simulink model "VFlexP"  (R2025a)
settings: Solver=ode23tb  StartTime=0.0  StopTime=40  FixedStep=5e-5
model workspace (MAT data in the model file):
  DCop_DCBUCK : object (value not decoded)
  Grid_CCVSC_idx = [2; 3; 4; 5; 6; 7; 8; 9; 10; 11; 12]
  Grid_CCVSCs = 1
  Grid_CCVSCs_buses = 1
  Grid_CCVSCs_toM = [0 1 0 0 0 0 0 0 0 0 0 0 ... (781 elements, 71x11)]
  Grid_C_Lines = [0.1 0.1 0.1 0.1]
  Grid_Cbuses = [0.05000002 0.10000002 0.10000002 0.10000002 0.05000002]
  Grid_DC : object (value not decoded)
  Grid_DCop_DCBUCK : object (value not decoded)
  Grid_DCop_DC_PES : object (value not decoded)
  Grid_DFIGs = 1
  Grid_DFIGs_buses = 1
  Grid_DGs : string (value not decoded)
  Grid_From_buses = [1 2 4 4]
  Grid_GFls = 1
  Grid_GFls_buses = 1
  Grid_GFr_idx = [1; 2; 3]
  Grid_GFrs = 1
  Grid_GFrs_buses = 1
  Grid_GFrs_toM = [1 0 0 0 0 0 0 0 0 1 0 0 ... (15 elements, 5x3)]
  Grid_IG_idx = 1
  Grid_IGs = 1
  Grid_IGs_buses = 1
  Grid_IGs_toM = [1; 0]
  Grid_L_Lines = [0.5 0.5 0.5 0.5]
  Grid_L_Loads = [0.000959999944704 0.000156249997559 0.00154855477548]
  Grid_Lines_fromM : object (value not decoded)
  Grid_Lines_toM : object (value not decoded)
  Grid_Load_buses = [2; 3; 4]
  Grid_Load_busesDC = []
  Grid_MGES_idx = [1; 2; 3]
  Grid_MGESs = 1
  Grid_MGESs_buses = [1; 5; 3]
  Grid_MGESs_toM = [1 0 0 0 0 0 0 0 0 1 0 0 ... (15 elements, 5x3)]
  Grid_MSGs = 1
  Grid_MSGs_buses = 1
  Grid_Nbuses = 5
  Grid_PQ_gen = [3; 2; 2]
  Grid_Ploads = [1250 4000 1250]
  Grid_PloadsDC = []
  Grid_Ps_lf = [0.274439537683 0.78 0.3]
  Grid_Qloads = [0.3 0.5 0.5]
  Grid_Qs_lf = [-0.0366071562958 0.126505596722 -0.0162964024532]
  Grid_R_Lines = [0.01 0.01 0.01 0.01]
  Grid_R_Loads = [3.9999997696 1.24999998047 3.8713869387]
  Grid_R_Loads_DC = 0
  Grid_Rcf = [50000000 50000000 50000000 50000000 50000000]
  Grid_SCs = 1
  Grid_SCs_buses = 1
  Grid_SG_idx = 1
  Grid_SGs = 1
  Grid_SGs_buses = 1
  Grid_SGs_toM = [1; 0]
  Grid_To_buses = [2 3 3 5]
  Grid_VCVSC_idx = [1; 2; 3; 4; 5; 6; 7; 8; 9; 10; 11; 12]
  Grid_VCVSCs = 1
  Grid_VCVSCs_buses = [1; 2; 3; 6; 8; 9; 12; 58; 59; 60; 63; 65]
  Grid_VCVSCs_toM = [1 0 0 0 0 0 0 0 0 0 0 0 ... (852 elements, 71x12)]
  Grid_VSM_idx = [1; 2; 3]
  Grid_VSMs = 1
  Grid_VSMs_buses = 1
  Grid_VSMs_toM = [1 0 0 0 0 0 0 0 0 1 0 0 ... (15 elements, 5x3)]
  Grid_admitt_matrix = [2.15353135314-19.7953135314i  -1.9801980198+19.801980198i; -1.9801980198+19.801980198i  2.15353135314-19.7953135314i]
  Grid_admitt_matrix_noloads = [1.98686468647-19.7953135314i  -1.9801980198+19.801980198i; -1.9801980198+19.801980198i  1.98686468647-19.7953135314i]
  Grid_bus = [1; 2; 6; 7; 8]
  Grid_busDC_complexity = [1 1 1]
  Grid_busDC_complexity_PF = [2 2 2]
  Grid_bus_complexity = [1 1 1 1 1]
  Grid_bus_complexity_PF = [1 1 1 1 1]
  Grid_buses_lf = [1; 5; 3]
  Grid_conductance_matrix = [100.00000002  -100  0; -100  200.00000002  -100; 0  -100  100.00000002]
  Grid_conductance_matrix_noloads = [100.00000002  -100  0; -100  200.00000002  -100; 0  -100  100.00000002]
  Grid_fref : object (value not decoded)
  Grid_gen_static_params : mBase (value not decoded)
  Grid_iPs_lf = [3.64378984326 1.28205128205 3.33333333333]
  Grid_iQs_lf = [-27.3170631425 7.90478860943 -61.3632366329]
  Grid_iadmitt_matrix = [2.88165849328-0.0982918688642i  2.87905051706-0.123273862303i; 2.87905051706-0.123273862303i  2.88165849328-0.0982918688642i]
  Grid_iadmitt_matrix_noloads = [37.5012524798-37.4874983544i  37.4987475202-37.5125016456i; 37.4987475202-37.5125016456i  37.5012524798-37.4874983544i]
  Grid_iconductance_matrix = [16666671.4556  16666671.4489  16666671.4456; 16666671.4489  16666671.4522  16666671.4489; 16666671.4456  16666671.4489  16666671.4556]
  Grid_iconductance_matrix_noloads = [16666671.4556  16666671.4489  16666671.4456; 16666671.4489  16666671.4522  16666671.4489; 16666671.4456  16666671.4489  16666671.4556]
  Grid_init_OK_bool = 1
  Grid_intconv_PF : object (value not decoded)
  Grid_lf_op : op_report (value not decoded)
  Grid_lineDC_complexity = [1 1]
  Grid_lineDC_complexity_PF = [2 2]
  Grid_line_complexity = [1 1 1 1]
  Grid_line_complexity_PF = [3 3 3 3]
  Grid_loadDC_complexity = []
  Grid_loadDC_complexity_PF = []
  Grid_load_complexity = [3 3 3]
  Grid_load_complexity_PF = [4 4 4]
  Grid_opDC_CCVSC : object (value not decoded)
  Grid_opDC_VSM : object (value not decoded)
  Grid_opGFr : object (value not decoded)
  Grid_opVCVSC : object (value not decoded)
  Grid_op_CCVSC : object (value not decoded)
  Grid_op_IG : object (value not decoded)
  Grid_op_MGES : object (value not decoded)
  Grid_op_SG : object (value not decoded)
  Grid_op_VSM : object (value not decoded)
  Grid_shift_lines = [0 0 0 0]
  Grid_tap_lines = [1 1 1 1]
  Grid_v_buses_mod = [1 1 1 0.9837920967 1]
  LinsysParamChangeStruct : Param1 (value not decoded)
  Lline = 0.01
  Rline = 1e-05
  linsys : object (value not decoded)
symbols that are objects in the model workspace (value not decoded): Grid_DCop_DC_PES, Grid_DCop_DCBUCK, Grid_op_CCVSC, Grid_op_IG, Grid_op_MGES, Grid_op_SG, Grid_op_VSM, Grid_opDC_CCVSC, Grid_opDC_VSM, Grid_opGFr, Grid_opVCVSC
undefined symbols (not defined in the file): block_buses_DC, block_idx, CCVSC_idx, Cf, costs, costs2, D, DFIGs_nodes, DiscIntNeverNeededParam, entity, Fb, Fi, From_nodes, grid_linsys, Grid_op_DFIG, Grid_op_DFIG_PQ, Grid_op_MSG, Grid_op_SC, Grid_op_VCVSC, H, initial_states_grid, K_1, K_3, K_5, K_A, K_C, K_IM, K_IR, K_P, K_PM, K_PR, K_S1, K_S2, K_S3, Ki_w, Kic, Kiv, Kp_id, Kp_theta, Kp_w, Kpc, Kpv, last_send, Lc, Lf, Lfd, Lkd1, Lkd2, Lkq1, Lkq2, Lkq3, Lmd, Lmq, Lsd, Lsq, m, M, Matrix_flux_to_i, mp, MSGs_buses ... (+44)
libraries: simulink x1048, eeGeneralControl x12
(part 11 of 50)

== system VFlexP/Grid/Generators/MSG/For Each Subsystem ==
  In1 : Inport  Partition=on  PartitionDimension=1  PartitionWidth=1  PartitionOffset=0
  Assignment : Assignment  DiagnosticForDimensions=Warning  IndexOptions=Index vector (dialog)  Indices=block_buses  OutputSizes=1
  For Each : ForEach  DisableCoverage=on
  Zero : Constant  Value=zeros(1,Nbuses)  VectorParams1D=off  OutDataTypeStr=Inherit: Inherit via back propagation
  Out1 : Outport  ConcatenationDimension=1
  wires:
  Assignment/1 -> Out1/1
  In1/1 -> Assignment/2
  Zero/1 -> Assignment/1

== system VFlexP/Grid/Generators/MSG/GRID CONVERTER CONTROL ==
  vd : Inport
  iad_ref : Inport  Port=2
  iad : Inport  Port=3
  iaq_ref : Inport  Port=4
  iaq : Inport  Port=5
  ws : Inport  Port=6
  PI Estator Current d : Subsystem
  PI Estator Current q : Subsystem
  Subsystem1 : Subsystem
  Subsystem3 : Subsystem
  Sum : Sum  Inputs=|+-
  Sum1 : Sum  Inputs=|+-
  vad : Outport  VectorParamsAs1DForOutWhenUnconnected=off
  vaq : Outport  Port=2  VectorParamsAs1DForOutWhenUnconnected=off
  wires:
  Subsystem1/1(vadq) -> vaq/1
  ws/1 -> Subsystem3/4(ws), Subsystem1/1(ws)
  iaq/1 -> Sum1/2, Subsystem3/3(iaq)
  iaq_ref/1 -> Sum1/1
  iad_ref/1 -> Sum/1
  Sum/1 -> PI Estator Current d/1(in)
  Sum1/1 -> PI Estator Current q/1(in)
  iad/1 -> Subsystem1/3(iad), Sum/2
  PI Estator Current d/1(out) -> Subsystem3/1(vad')
  PI Estator Current q/1(out) -> Subsystem1/2(vaq')
  vd/1 -> Subsystem3/2(vd)
  Subsystem3/1(vad) -> vad/1

== system VFlexP/Grid/Generators/MSG/MACHINE CONVERTER CONTROL ==
  isd_ref : Inport
  isd : Inport  Port=2
  isq_ref : Inport  Port=3
  isq : Inport  Port=4
  wr : Inport  Port=5
  ifd : Inport  Port=6
  PI Estator Current d : Subsystem
  PI Estator Current q : Subsystem
  Subsystem1 : Subsystem
  Subsystem3 : Subsystem
  Sum : Sum  Inputs=|+-
  Sum1 : Sum  Inputs=|+-
  vsd : Outport  VectorParamsAs1DForOutWhenUnconnected=off
  vsq : Outport  Port=2  VectorParamsAs1DForOutWhenUnconnected=off
  wires:
  wr/1 -> Subsystem3/3(wr), Subsystem1/1(wr)
  isq/1 -> Sum1/2, Subsystem3/2(isq)
  isq_ref/1 -> Sum1/1
  isd_ref/1 -> Sum/1
  Sum/1 -> PI Estator Current d/1(in)
  Sum1/1 -> PI Estator Current q/1(in)
  isd/1 -> Subsystem1/3(isd), Sum/2
  PI Estator Current q/1(out) -> Subsystem1/2(vsq')
  Subsystem3/1(vsd) -> vsd/1
  ifd/1 -> Subsystem1/4(ifd)
  PI Estator Current d/1(out) -> Subsystem3/1(vsd')
  Subsystem1/1(vsq) -> vsq/1

== system VFlexP/Grid/Generators/MSG/Reference frame transform3 ==
  in_d : Inport
  theta : Inport  Port=2
  in_q : Inport  Port=3
  Complex to Real-Imag : ComplexToRealImag
  Cos : Trigonometry  SCDEnableBlockLinearizationSpecification=on  Operator=cos
  Product : Product
  Real-Imag to Complex : RealImagToComplex
  Real-Imag to Complex1 : RealImagToComplex
  Sin : Trigonometry  SCDEnableBlockLinearizationSpecification=on
  out_d : Outport
  out_q : Outport  Port=2
  wires:
  Complex to Real-Imag/2 -> out_q/1
  Real-Imag to Complex1/1 -> Product/1
  Real-Imag to Complex/1 -> Product/2
  Product/1 -> Complex to Real-Imag/1
  theta/1 -> Sin/1, Cos/1
  Cos/1 -> Real-Imag to Complex1/1
  Sin/1 -> Real-Imag to Complex1/2
  Complex to Real-Imag/1 -> out_d/1
  in_q/1 -> Real-Imag to Complex/2
  in_d/1 -> Real-Imag to Complex/1

== system VFlexP/Grid/Generators/MSG/Reference frame transform5 ==
  in_d : Inport
  theta : Inport  Port=2
  in_q : Inport  Port=3
  Complex to Real-Imag : ComplexToRealImag
  Cos : Trigonometry  SCDEnableBlockLinearizationSpecification=on  Operator=cos
  Product : Product
  Real-Imag to Complex : RealImagToComplex
  Real-Imag to Complex1 : RealImagToComplex
  Sin : Trigonometry  SCDEnableBlockLinearizationSpecification=on
  out_d : Outport
  out_q : Outport  Port=2
  wires:
  in_d/1 -> Real-Imag to Complex/1
  in_q/1 -> Real-Imag to Complex/2
  Complex to Real-Imag/1 -> out_d/1
  Sin/1 -> Real-Imag to Complex1/2
  Cos/1 -> Real-Imag to Complex1/1
  theta/1 -> Cos/1, Sin/1
  Product/1 -> Complex to Real-Imag/1
  Real-Imag to Complex/1 -> Product/2
  Real-Imag to Complex1/1 -> Product/1
  Complex to Real-Imag/2 -> out_q/1

== system VFlexP/Grid/Generators/MSG/Rotor axis ==
  te : Inport
  tm : Inport  Port=2
  Gain : Gain  Gain=1/2./H
  Gain1 : Gain  Gain=D
  Sum1 : Sum  Inputs=-|+|-  InputSameDT=on  SaturateOnIntegerOverflow=on  OutDataTypeStr=Inherit: Same as first input
  \omega_r : Integrator  InitialCondition=Grid_op_MSG.op.States(5).x'  UpperSaturationLimit=2*pi  LowerSaturationLimit=0
  wr : Outport  VectorParamsAs1DForOutWhenUnconnected=off
  wires:
  Gain1/1 -> Sum1/3
  Gain/1 -> \omega_r/1
  Sum1/1 -> Gain/1
  te/1 -> Sum1/2
  \omega_r/1 -> Gain1/1, wr/1
  tm/1 -> Sum1/1

== system VFlexP/Grid/Generators/MSG/Stator circuit MSG ==
  vsd : Inport
  vsq : Inport  Port=2
  i : Inport  Port=3
  ws : Inport  Port=4
  vfd : Inport  Port=5
  vad : Inport  Port=6
  vaq : Inport  Port=7
  vd : Inport  Port=8
  vq : Inport  Port=9
  wr : Inport  Port=10
  Gain1 : Gain  Gain=Rs_pu
  Gain{4..6,17} (4 alike) : Gain  Gain=-1
  Gain2 : Gain  Gain=Rs_pu
  Gain3 : Gain  Gain=Rfd_pu
  Matrix Concatenate : Concatenate  NumInputs=6  Mode=Multidimensional array
  Product{1..5} (5 alike) : Product
  Selector : Selector  NumberOfDimensions=2  InputPortWidth=9  IndexOptions=Index vector (dialog),Select all  Indices=[1],1  OutputSizes=1,1
  Selector1 : Selector  NumberOfDimensions=2  InputPortWidth=9  IndexOptions=Index vector (dialog),Select all  Indices=[2],1  OutputSizes=1,1
  Selector2 : Selector  NumberOfDimensions=2  InputPortWidth=9  IndexOptions=Index vector (dialog),Select all  Indices=5,1  OutputSizes=1,1
  Selector3 : Selector  NumberOfDimensions=2  InputPortWidth=9  IndexOptions=Index vector (dialog),Select all  Indices=[4],1  OutputSizes=1,1
  Selector4 : Selector  InputPortWidth=length(fref.ref_units)  IndexOptions=Index vector (dialog)  Indices=block_fref  OutputSizes=1
  Selector9 : Selector  NumberOfDimensions=2  InputPortWidth=9  IndexOptions=Index vector (dialog),Select all  Indices=6,1  OutputSizes=1,1
  Subsystem2 : Subsystem
  Sum : Sum  Inputs=++|
  Sum1 : Sum  Inputs=-|+|-  InputSameDT=on  SaturateOnIntegerOverflow=on  OutDataTypeStr=Inherit: Same as first input
  Sum2 : Sum  Inputs=-|+|-  InputSameDT=on  SaturateOnIntegerOverflow=on  OutDataTypeStr=Inherit: Same as first input
  Zero2 : Constant  Value=zeros(1, length(MSGs_buses))  VectorParams1D=off  OutDataTypeStr=Inherit: Inherit via back propagation
  psifd : Integrator  InitialCondition=Grid_op_MSG.op.States(8).x'
  psis_d : Integrator  InitialCondition=Grid_op_MSG.op.States(9).x'
  psis_q : Integrator  InitialCondition=Grid_op_MSG.op.States(10).x'
  psi : Outport  VectorParamsAs1DForOutWhenUnconnected=off
  wires:
  Product4/1 -> psis_q/1
  Sum1/1 -> Product4/1
  Gain3/1 -> Sum/2
  vfd/1 -> Sum/1
  Sum/1 -> Product5/2
  psifd/1 -> Matrix Concatenate/4
  Matrix Concatenate/1 -> psi/1
  Product5/1 -> psifd/1
  Zero2/1 -> Matrix Concatenate/3
  vsd/1 -> Sum2/2
  Sum2/1 -> Product3/2
  Product3/1 -> psis_d/1
  Gain17/1 -> Product1/2
  psis_q/1 -> Matrix Concatenate/2, Gain17/1  "psis_q"
  Product1/1 -> Sum2/1
  Product2/1 -> Sum1/3
  psis_d/1 -> Product2/1, Matrix Concatenate/1
  Gain2/1 -> Sum2/3
  Gain1/1 -> Sum1/1
  vsq/1 -> Sum1/2
  Selector9/1 -> Subsystem2/4(iq)  "iaq"
  Selector2/1 -> Subsystem2/3(id)  "iad"
  vad/1 -> Subsystem2/1(vad)
  Subsystem2/1(d) -> Matrix Concatenate/5
  Subsystem2/2(q) -> Matrix Concatenate/6
  vaq/1 -> Subsystem2/2(vaq)
  [ws] -> Subsystem2/5(ws)
  wr/1 -> Product1/1, Product2/2
  vq/1 -> Subsystem2/7(vq)
  vd/1 -> Subsystem2/6(vd)
  ws/1 -> [ws]
  i/1 -> Gain6/1
  Selector/1 -> Gain2/1
  Selector1/1 -> Gain1/1
  Gain4/1 -> Selector2/1
  Gain5/1 -> Selector9/1
  Selector3/1 -> Gain3/1  "ifd"
  Gain6/1 -> Gain5/1, Gain4/1, Selector/1, Selector1/1, Selector3/1
  Selector4/1 -> Product4/2, Product5/1, Product3/1
  [omega_base] -> Selector4/1

== system VFlexP/Grid/Generators/MSG/Subsystem ==
  wref : Inport
  wr : Inport  Port=2
  PI omega : Subsystem
  Sum : Sum  Inputs=|+-
  isq_ref : Outport
  wires:
  PI omega/1(out) -> isq_ref/1
  Sum/1 -> PI omega/1(in)
  wref/1 -> Sum/1
  wr/1 -> Sum/2

== system VFlexP/Grid/Generators/MSG/Torque ==
  psi : Inport
  isd : Inport  Port=2
  isq : Inport  Port=3
  Product1 : Product
  Product2 : Product
  Selector : Selector  NumberOfDimensions=2  InputPortWidth=9  IndexOptions=Index vector (dialog),Select all  Indices=[1],1  OutputSizes=1,1
  Selector1 : Selector  NumberOfDimensions=2  InputPortWidth=9  IndexOptions=Index vector (dialog),Select all  Indices=[2],1  OutputSizes=1,1
  Sum : Sum  Inputs=+||-
  te : Outport  VectorParamsAs1DForOutWhenUnconnected=off
  wires:
  Product1/1 -> Sum/1
  Sum/1 -> te/1
  Selector/1 -> Product1/1  "psistatordq"
  psi/1 -> Selector1/1, Selector/1
  Product2/1 -> Sum/2
  isq/1 -> Product1/2
  isd/1 -> Product2/1
  Selector1/1 -> Product2/2  "psistatordq"

== system VFlexP/Grid/Generators/MSG/Vc control ==
  Vc_2_ref : Inport
  vsd : Inport  Port=2
  vsq : Inport  Port=3
  isd : Inport  Port=4
  isq : Inport  Port=5
  vad : Inport  Port=6
  vaq : Inport  Port=7
  iad : Inport  Port=8
  iaq : Inport  Port=9
  Gain : Gain  Gain=2./Cf_pu
  PI Vc2 : Subsystem
  Product{1..2,5..6} (4 alike) : Product
  Scope : Scope
      settings: ActiveDisplayYMinimum=0.13056  ActiveDisplayYMaximum=1.2418  DataLoggingVariableName=ScopeData2
  Sum : Sum  Inputs=|+-
  Sum1 : Sum  Inputs=|++
  Sum2 : Sum  Inputs=+-|
  Sum4 : Sum  Inputs=|++
  Vc : Integrator  InitialCondition=Grid_op_MSG.op.States(13).x'
  iad_ref : Outport  VectorParamsAs1DForOutWhenUnconnected=off
  wires:
  Sum1/1 -> Sum2/2  "pa"
  Product1/1 -> Sum1/1
  Product2/1 -> Sum1/2
  vad/1 -> Product1/1
  vaq/1 -> Product2/1
  iaq/1 -> Product2/2
  iad/1 -> Product1/2
  Sum4/1 -> Sum2/1  "ps"
  isd/1 -> Product5/2
  isq/1 -> Product6/2
  vsq/1 -> Product6/1
  vsd/1 -> Product5/1
  Product6/1 -> Sum4/2
  Product5/1 -> Sum4/1
  Sum/1 -> PI Vc2/1(in)
  PI Vc2/1(out) -> iad_ref/1
  Sum2/1 -> Gain/1
  Vc/1 -> Scope/1, Sum/2
  Gain/1 -> Vc/1
  Vc_2_ref/1 -> Sum/1

== system VFlexP/Grid/Generators/MSG/connect ==
  id : Inport
  iq : Inport  Port=2
  connect : Inport  Port=3
  Switch : Switch  Criteria=u2 > Threshold  ZeroCross=off  SaturateOnIntegerOverflow=off  InputSameDT=off
  Switch1 : Switch  Criteria=u2 > Threshold  ZeroCross=off  SaturateOnIntegerOverflow=off  InputSameDT=off
  Zero1 : Constant  Value=0  VectorParams1D=off  OutDataTypeStr=Inherit: Inherit via back propagation
  Zero2 : Constant  Value=0  VectorParams1D=off  OutDataTypeStr=Inherit: Inherit via back propagation
  id_real : Outport
  iq_real : Outport  Port=2
  connected : Outport  Port=3  OutDataTypeStr=boolean
  wires:
  Switch/1 -> id_real/1
  Zero1/1 -> Switch/3
  id/1 -> Switch/1
  connect/1 -> connected/1, Switch1/2, Switch/2
  Switch1/1 -> iq_real/1
  iq/1 -> Switch1/1
  Zero2/1 -> Switch1/3

== system VFlexP/Grid/Generators/MSG/psi->i ==
  psi : Inport
  Display : Display
  Gain : Gain  Gain=Lbiginv  Multiplication=Matrix(K*u)
  Reshape_in : Reshape  OutputDimensionality=Column vector (2-D)
  Reshape_out : Reshape  OutputDimensionality=Customize  OutputDimensions=[6, length(MSGs_buses)]
  Selector : Selector  NumberOfDimensions=2  InputPortWidth=9  IndexOptions=Index vector (dialog),Select all  Indices=[1],1  OutputSizes=1,1
  Selector1 : Selector  NumberOfDimensions=2  InputPortWidth=9  IndexOptions=Index vector (dialog),Select all  Indices=[2],1  OutputSizes=1,1
  Selector2 : Selector  NumberOfDimensions=2  InputPortWidth=9  IndexOptions=Index vector (dialog),Select all  Indices=5,1  OutputSizes=1,1
  Selector3 : Selector  NumberOfDimensions=2  InputPortWidth=9  IndexOptions=Index vector (dialog),Select all  Indices=6,1  OutputSizes=1,1
  Selector4 : Selector  NumberOfDimensions=2  InputPortWidth=9  IndexOptions=Index vector (dialog),Select all  Indices=4,1  OutputSizes=1,1
  Selector5 : Selector  NumberOfDimensions=2  InputPortWidth=9  IndexOptions=Index vector (dialog),Select all  Indices=3,1  OutputSizes=1,1
  isd : Outport  VectorParamsAs1DForOutWhenUnconnected=off
  i : Outport  Port=2  VectorParamsAs1DForOutWhenUnconnected=off
  isq : Outport  Port=3  VectorParamsAs1DForOutWhenUnconnected=off
  ifd : Outport  Port=4  VectorParamsAs1DForOutWhenUnconnected=off
  iad : Outport  Port=5  VectorParamsAs1DForOutWhenUnconnected=off
  iaq : Outport  Port=6  VectorParamsAs1DForOutWhenUnconnected=off
  wires:
  Selector/1 -> isd/1
  Gain/1 -> Reshape_out/1
  psi/1 -> Reshape_in/1
  Reshape_in/1 -> Gain/1
  Selector1/1 -> isq/1
  Selector4/1 -> ifd/1
  Selector2/1 -> iad/1
  Selector3/1 -> iaq/1
  Reshape_out/1 -> Selector2/1, Selector4/1, i/1, Selector/1, Selector1/1, Selector5/1, Selector3/1
  Selector5/1 -> Display/1

== system VFlexP/Grid/Generators/MSG/trim_output ==
  id : Inport
  iq : Inport  Port=2
  vd : Inport  Port=3
  vq : Inport  Port=4
  Out1 : Outport
  Out2 : Outport  Port=2
  Out3 : Outport  Port=3
  Out4 : Outport  Port=4
  wires:
  id/1 -> Out1/1
  vq/1 -> Out4/1
  vd/1 -> Out3/1
  iq/1 -> Out2/1

== system VFlexP/Grid/Generators/SC/AVR_Exciter ==
  in : Inport
  Gain : Gain  Gain=1/T_s
  Sum4 : Sum  Inputs=|+-
  x_a : Integrator  InitialCondition=Grid_op_SC.op.States(1).x'
  out : Outport
  wires:
  Gain/1 -> x_a/1
  Sum4/1 -> Gain/1
  in/1 -> Sum4/1
  x_a/1 -> out/1, Sum4/2

== system VFlexP/Grid/Generators/SC/AVR_LeadLag ==
  In1 : Inport
  Gain : Gain  Gain=1/T_1
  Gain2 : Gain  Gain=T_2/T_1
  Sum : Sum  Inputs=|+-
  Sum1 : Sum  Inputs=++|
  x_f : Integrator  InitialCondition=Grid_op_SC.op.States(2).x'
  Out1 : Outport
  wires:
  x_f/1 -> Sum1/2, Sum/2
  Gain/1 -> x_f/1
  Sum/1 -> Gain/1, Gain2/1
  Gain2/1 -> Sum1/1
  Sum1/1 -> Out1/1
  In1/1 -> Sum/1

== system VFlexP/Grid/Generators/SC/AVR_MainRegulator ==
  in : Inport
  Gain : Gain  Gain=1/T_s
  Sum4 : Sum  Inputs=|+-
  x_a : Integrator  InitialCondition=Grid_op_SC.op.States(3).x'
  out : Outport
  wires:
  in/1 -> Sum4/1
  x_a/1 -> Sum4/2, out/1
  Sum4/1 -> Gain/1
  Gain/1 -> x_a/1

== system VFlexP/Grid/Generators/SC/AVR_Vmeas_Filter ==
  in : Inport
  Gain : Gain  Gain=1/T_r
  Sum4 : Sum  Inputs=|+-
  x_a : Integrator  InitialCondition=Grid_op_SC.op.States(4).x'
  out : Outport
  wires:
  Gain/1 -> x_a/1
  Sum4/1 -> Gain/1
  in/1 -> Sum4/1
  x_a/1 -> out/1, Sum4/2

== system VFlexP/Grid/Generators/SC/For Each Subsystem ==
  In1 : Inport  Partition=on  PartitionDimension=1  PartitionWidth=1  PartitionOffset=0
  For Each : ForEach  DisableCoverage=on
  Gen_To : MATLAB Function  TreatAsAtomicUnit=on
  Out1 : Outport  ConcatenationDimension=1
  wires:
  Gen_To/1(y) -> Out1/1
  In1/1 -> Gen_To/1(u)

== system VFlexP/Grid/Generators/SC/Reference frame transform1 ==
  in_d : Inport
  theta : Inport  Port=2
  in_q : Inport  Port=3
  Complex to Real-Imag : ComplexToRealImag
  Cos : Trigonometry  SCDEnableBlockLinearizationSpecification=on  Operator=cos
  Product : Product
  Real-Imag to Complex : RealImagToComplex
  Real-Imag to Complex1 : RealImagToComplex
  Sin : Trigonometry  SCDEnableBlockLinearizationSpecification=on
  out_d : Outport
  out_q : Outport  Port=2
  wires:
  in_d/1 -> Real-Imag to Complex/1
  in_q/1 -> Real-Imag to Complex/2
  Complex to Real-Imag/1 -> out_d/1
  Sin/1 -> Real-Imag to Complex1/2
  Cos/1 -> Real-Imag to Complex1/1
  theta/1 -> Cos/1, Sin/1
  Product/1 -> Complex to Real-Imag/1
  Real-Imag to Complex/1 -> Product/2
  Real-Imag to Complex1/1 -> Product/1
  Complex to Real-Imag/2 -> out_q/1

== system VFlexP/Grid/Generators/SC/Reference frame transform2 ==
  in_d : Inport
  theta : Inport  Port=2
  in_q : Inport  Port=3
  Complex to Real-Imag : ComplexToRealImag
  Cos : Trigonometry  SCDEnableBlockLinearizationSpecification=on  Operator=cos
  Product : Product
  Real-Imag to Complex : RealImagToComplex
  Real-Imag to Complex1 : RealImagToComplex
  Sin : Trigonometry  SCDEnableBlockLinearizationSpecification=on
  out_d : Outport
  out_q : Outport  Port=2
  wires:
  in_d/1 -> Real-Imag to Complex/1
  in_q/1 -> Real-Imag to Complex/2
  Complex to Real-Imag/1 -> out_d/1
  Sin/1 -> Real-Imag to Complex1/2
  Cos/1 -> Real-Imag to Complex1/1
  theta/1 -> Cos/1, Sin/1
  Product/1 -> Complex to Real-Imag/1
  Real-Imag to Complex/1 -> Product/2
  Real-Imag to Complex1/1 -> Product/1
  Complex to Real-Imag/2 -> out_q/1

== system VFlexP/Grid/Generators/SC/Rotor axis ==
  te : Inport
  tm : Inport  Port=2
  Gain : Gain  Gain=1/2./H
  Gain1 : Gain  Gain=D
  Sum1 : Sum  Inputs=+|-|-  InputSameDT=on  SaturateOnIntegerOverflow=on  OutDataTypeStr=Inherit: Same as first input
  \omega_r : Integrator  InitialCondition=Grid_op_SC.op.States(8).x'  UpperSaturationLimit=2*pi  LowerSaturationLimit=0
  wr : Outport  VectorParamsAs1DForOutWhenUnconnected=off
  wires:
  tm/1 -> Sum1/1
  \omega_r/1 -> wr/1, Gain1/1
  te/1 -> Sum1/2
  Sum1/1 -> Gain/1
  Gain/1 -> \omega_r/1
  Gain1/1 -> Sum1/3

== system VFlexP/Grid/Generators/SC/Stator circuit ==
  vsd : Inport
  vsq : Inport  Port=2
  i : Inport  Port=3
  ws : Inport  Port=4
  vfd : Inport  Port=5
  Gain1 : Gain  Gain=Rs_pu
  Gain17 : Gain  Gain=-1
  Gain2 : Gain  Gain=Rs_pu
  Gain3 : Gain  Gain=Rfd_pu
  Gain4 : Gain  Gain=Rkd1_pu
  Gain5 : Gain  Gain=Rkd2_pu
  Gain6 : Gain  Gain=Rkq1_pu
  Gain7 : Gain  Gain=Rkq2_pu
  Gain8 : Gain  Gain=Rkq3_pu
  Gain9 : Gain  Gain=-1
  Matrix Concatenate : Concatenate  NumInputs=9  Mode=Multidimensional array
  Product{1..10} (10 alike) : Product
  Selector : Selector  NumberOfDimensions=2  InputPortWidth=9  IndexOptions=Index vector (dialog),Select all  Indices=[1],1  OutputSizes=1,1
  Selector1 : Selector  NumberOfDimensions=2  InputPortWidth=9  IndexOptions=Index vector (dialog),Select all  Indices=[2],1  OutputSizes=1,1
  Selector2 : Selector  InputPortWidth=length(fref.ref_units)  IndexOptions=Index vector (dialog)  Indices=block_fref  OutputSizes=1
  Selector3 : Selector  NumberOfDimensions=2  InputPortWidth=9  IndexOptions=Index vector (dialog),Select all  Indices=[4],1  OutputSizes=1,1
  Selector4 : Selector  NumberOfDimensions=2  InputPortWidth=9  IndexOptions=Index vector (dialog),Select all  Indices=[5],1  OutputSizes=1,1
  Selector5 : Selector  NumberOfDimensions=2  InputPortWidth=9  IndexOptions=Index vector (dialog),Select all  Indices=[6],1  OutputSizes=1,1
  Selector6 : Selector  NumberOfDimensions=2  InputPortWidth=9  IndexOptions=Index vector (dialog),Select all  Indices=[7],1  OutputSizes=1,1
  Selector7 : Selector  NumberOfDimensions=2  InputPortWidth=9  IndexOptions=Index vector (dialog),Select all  Indices=[8],1  OutputSizes=1,1
  Selector8 : Selector  NumberOfDimensions=2  InputPortWidth=9  IndexOptions=Index vector (dialog),Select all  Indices=[9],1  OutputSizes=1,1
  Sum : Sum  Inputs=++|
  Sum1 : Sum  Inputs=-|+|-  InputSameDT=on  SaturateOnIntegerOverflow=on  OutDataTypeStr=Inherit: Same as first input
  Sum2 : Sum  Inputs=-|+|-  InputSameDT=on  SaturateOnIntegerOverflow=on  OutDataTypeStr=Inherit: Same as first input
  Zero1 : Constant  Value=zeros(1, length(block_buses))  VectorParams1D=off  OutDataTypeStr=Inherit: Inherit via back propagation
  psifd : Integrator  InitialCondition=Grid_op_SC.op.States(9).x'
  psikd1 : Integrator  InitialCondition=Grid_op_SC.op.States(10).x'
  psikd2 : Integrator  InitialCondition=Grid_op_SC.op.States(11).x'
  psikq1 : Integrator  InitialCondition=Grid_op_SC.op.States(12).x'
  psikq2 : Integrator  InitialCondition=Grid_op_SC.op.States(13).x'
  psikq3 : Integrator  InitialCondition=Grid_op_SC.op.States(14).x'
  psis_d : Integrator  InitialCondition=Grid_op_SC.op.States(15).x'
  psis_q : Integrator  InitialCondition=Grid_op_SC.op.States(16).x'
  psi : Outport  VectorParamsAs1DForOutWhenUnconnected=off
  wires:
  Product3/1 -> psis_q/1
  Sum1/1 -> Product3/1
  Selector3/1 -> Gain3/1  "ifd"
  Selector8/1 -> Gain8/1  "ikq3"
  Selector7/1 -> Gain7/1  "ikq2"
  Selector6/1 -> Gain6/1  "ikq1"
  Selector5/1 -> Gain5/1  "ikd2"
  Selector4/1 -> Gain4/1  "ikd1"
  Gain3/1 -> Sum/2
  vfd/1 -> Sum/1
  Sum/1 -> Product5/2
  Gain4/1 -> Product6/2
  Gain6/1 -> Product8/2
  Gain8/1 -> Product10/2
  Gain7/1 -> Product9/2
  psikd2/1 -> Matrix Concatenate/6
  psifd/1 -> Matrix Concatenate/4
  psikq3/1 -> Matrix Concatenate/9
  psikq1/1 -> Matrix Concatenate/7
  psikd1/1 -> Matrix Concatenate/5
  Matrix Concatenate/1 -> psi/1
  i/1 -> Gain9/1
  Product5/1 -> psifd/1
  Product6/1 -> psikd1/1
  Product7/1 -> psikd2/1
  Product8/1 -> psikq1/1
  Product9/1 -> psikq2/1
  Product10/1 -> psikq3/1
  Gain9/1 -> Selector8/1, Selector7/1, Selector6/1, Selector5/1, Selector4/1, Selector1/1, Selector/1, Selector3/1
  psikq2/1 -> Matrix Concatenate/8
  Zero1/1 -> Matrix Concatenate/3
  vsd/1 -> Sum2/2
  Sum2/1 -> Product4/2
  Product4/1 -> psis_d/1
  ws/1 -> Product1/1, Product2/2
  Gain17/1 -> Product1/2
  psis_q/1 -> Matrix Concatenate/2, Gain17/1  "psis_q"
  Product1/1 -> Sum2/1
  Product2/1 -> Sum1/3
  psis_d/1 -> Product2/1, Matrix Concatenate/1
  Selector/1 -> Gain2/1
  Gain2/1 -> Sum2/3
  Selector1/1 -> Gain1/1
  Gain1/1 -> Sum1/1
  vsq/1 -> Sum1/2
  [omega_base] -> Selector2/1
  Selector2/1 -> Product10/1, Product9/1, Product8/1, Product7/1, Product6/1, Product5/1, Product4/1, Product3/2
  Gain5/1 -> Product7/2

== system VFlexP/Grid/Generators/SC/Torque ==
  psi : Inport
  isd : Inport  Port=2
  isq : Inport  Port=3
  Product1 : Product
  Product2 : Product
  Selector : Selector  NumberOfDimensions=2  InputPortWidth=9  IndexOptions=Index vector (dialog),Select all  Indices=[1],1  OutputSizes=1,1
  Selector1 : Selector  NumberOfDimensions=2  InputPortWidth=9  IndexOptions=Index vector (dialog),Select all  Indices=[2],1  OutputSizes=1,1
  Sum : Sum  Inputs=+||-
  te : Outport  VectorParamsAs1DForOutWhenUnconnected=off
  wires:
  Product1/1 -> Sum/1
  Sum/1 -> te/1
  Selector/1 -> Product1/1  "psistatordq"
  psi/1 -> Selector1/1, Selector/1
  Product2/1 -> Sum/2
  isq/1 -> Product1/2
  isd/1 -> Product2/1
  Selector1/1 -> Product2/2  "psistatordq"

== system VFlexP/Grid/Generators/SC/connect ==
  id : Inport
  iq : Inport  Port=2
  connect : Inport  Port=3
  Switch : Switch  Criteria=u2 > Threshold  ZeroCross=off  SaturateOnIntegerOverflow=off  InputSameDT=off
  Switch1 : Switch  Criteria=u2 > Threshold  ZeroCross=off  SaturateOnIntegerOverflow=off  InputSameDT=off
  Zero1 : Constant  Value=0  VectorParams1D=off  OutDataTypeStr=Inherit: Inherit via back propagation
  Zero2 : Constant  Value=0  VectorParams1D=off  OutDataTypeStr=Inherit: Inherit via back propagation
  id_real : Outport
  iq_real : Outport  Port=2
  connected : Outport  Port=3  OutDataTypeStr=boolean
  wires:
  Switch/1 -> id_real/1
  Zero1/1 -> Switch/3
  id/1 -> Switch/1
  connect/1 -> connected/1, Switch1/2, Switch/2
  Switch1/1 -> iq_real/1
  iq/1 -> Switch1/1
  Zero2/1 -> Switch1/3

== system VFlexP/Grid/Generators/SC/psi->i ==
  psi : Inport
  Gain : Gain  Gain=Lbiginv  Multiplication=Matrix(K*u)
  Reshape_in : Reshape  OutputDimensionality=Column vector (2-D)
  Reshape_out : Reshape  OutputDimensionality=Customize  OutputDimensions=[9, length(SCs_buses)]
  Selector : Selector  NumberOfDimensions=2  InputPortWidth=9  IndexOptions=Index vector (dialog),Select all  Indices=[1],1  OutputSizes=1,1
  Selector1 : Selector  NumberOfDimensions=2  InputPortWidth=9  IndexOptions=Index vector (dialog),Select all  Indices=[2],1  OutputSizes=1,1
  isd : Outport  VectorParamsAs1DForOutWhenUnconnected=off
  i : Outport  Port=2  VectorParamsAs1DForOutWhenUnconnected=off
  isq : Outport  Port=3  VectorParamsAs1DForOutWhenUnconnected=off
  wires:
  Selector/1 -> isd/1
  Gain/1 -> Reshape_out/1
  psi/1 -> Reshape_in/1
  Reshape_in/1 -> Gain/1
  Reshape_out/1 -> Selector1/1, Selector/1, i/1
  Selector1/1 -> isq/1

== system VFlexP/Grid/Generators/SC/trim_output ==
  id : Inport
  iq : Inport  Port=2
  vd : Inport  Port=3
  vq : Inport  Port=4
  Out1 : Outport
  Out2 : Outport  Port=2
  Out3 : Outport  Port=3
  Out4 : Outport  Port=4
  wires:
  id/1 -> Out1/1
  vq/1 -> Out4/1
  vd/1 -> Out3/1
  iq/1 -> Out2/1

== system VFlexP/Grid/Generators/SG/AVR_Exciter ==
  in : Inport
  Gain : Gain  Gain=1/T_s
  Sum4 : Sum  Inputs=|+-
  x_a : Integrator  InitialCondition=Grid_op_SG.op.States(1).x'
  out : Outport
  wires:
  Gain/1 -> x_a/1
  Sum4/1 -> Gain/1
  in/1 -> Sum4/1
  x_a/1 -> out/1, Sum4/2

== system VFlexP/Grid/Generators/SG/AVR_LeadLag ==
  In1 : Inport
  Gain : Gain  Gain=1/T_1
  Gain2 : Gain  Gain=T_2/T_1
  Sum : Sum  Inputs=|+-
  Sum1 : Sum  Inputs=++|
  x_f : Integrator  InitialCondition=Grid_op_SG.op.States(2).x'
  Out1 : Outport
  wires:
  x_f/1 -> Sum1/2, Sum/2
  Gain/1 -> x_f/1
  Sum/1 -> Gain/1, Gain2/1
  Gain2/1 -> Sum1/1
  Sum1/1 -> Out1/1
  In1/1 -> Sum/1

== system VFlexP/Grid/Generators/SG/AVR_MainRegulator ==
  in : Inport
  Gain : Gain  Gain=1/T_s
  Sum4 : Sum  Inputs=|+-
  x_a : Integrator  InitialCondition=Grid_op_SG.op.States(3).x'
  out : Outport
  wires:
  in/1 -> Sum4/1
  x_a/1 -> Sum4/2, out/1
  Sum4/1 -> Gain/1
  Gain/1 -> x_a/1

== system VFlexP/Grid/Generators/SG/AVR_Vmeas_Filter ==
  in : Inport
  Gain : Gain  Gain=1/T_r
  Sum4 : Sum  Inputs=|+-
  x_a : Integrator  InitialCondition=Grid_op_SG.op.States(4).x'
  out : Outport
  wires:
  Gain/1 -> x_a/1
  Sum4/1 -> Gain/1
  in/1 -> Sum4/1
  x_a/1 -> out/1, Sum4/2

== system VFlexP/Grid/Generators/SG/AVR_Vmeas_Filter1 ==
  in : Inport
  Gain : Gain  Gain=1/T_r
  Sum4 : Sum  Inputs=|+-
  x_a : Integrator  InitialCondition=Grid_op_SG.op.States(4).x'
  out : Outport
  wires:
  x_a/1 -> Sum4/2, out/1
  in/1 -> Sum4/1
  Sum4/1 -> Gain/1
  Gain/1 -> x_a/1

== system VFlexP/Grid/Generators/SG/AVR_Vmeas_Filter2 ==
  in : Inport
  Gain : Gain  Gain=1/T_r
  Sum4 : Sum  Inputs=|+-
  x_a : Integrator  InitialCondition=Grid_op_SG.op.States(5).x'
  out : Outport
  wires:
  Gain/1 -> x_a/1
  Sum4/1 -> Gain/1
  in/1 -> Sum4/1
  x_a/1 -> out/1, Sum4/2

== system VFlexP/Grid/Generators/SG/Electromagnetic ==
  note: 1) Add Subsystem or Model blocks as valid variant choices.
      | 2) You cannot connect blocks at this level. At simulation, connectivity is automatically
      | determined, based on the active variant and port name matching.
  vsd : Inport
  vsq : Inport  Port=2
  vfd : Inport  Port=3
  ws : Inport  Port=4
  order 2 : Subsystem  VariantControl=order 2
  order 8 : Subsystem  VariantControl=order 8
  order 8 nomatrix : Subsystem  VariantControl=order 1  mask{Lssd_pu=Lssd_pu, Lssq_pu=Lssq_pu, Lmd_pu=Lmd_pu, Lmq_pu=Lmq_pu, Lfd_pu=Lfd_pu, Lkd1_pu=Lkd1_pu, Lkd2_pu=Lkd2_pu, Lkq1_pu=Lkq1_pu, Lkq2_pu=Lkq2_pu, Lkq3_pu=Lkq3_pu}
      mask init:
      | for i=1:length(Lssd_pu)
      |         Lssd = Lssd_pu(i);
      |         Lssq = Lssq_pu(i);
      |         Lmd = Lmd_pu(i);
      |         Lmq = Lmq_pu(i);
      |         Lfd = Lfd_pu(i);
      |         Lkd1 = Lkd1_pu(i);
      |         Lkd2 = Lkd2_pu(i);
      |         Lkq1 = Lkq1_pu(i);
      |         Lkq2 = Lkq2_pu(i);
      |         Lkq3 = Lkq3_pu(i);
      |         Matrix_flux_to_i(:,:,i) = [(0 - (Lfd(i)*Lmd(i)^2 + Lkd2(i)*Lmd(i)^2 - Lmd(i)^3 - Lfd(i)*Lkd1(i)*Lkd2(i))/(2*Lmd(i)^4 - Lkd1(i)*Lmd(i)^3 - 2*Lkd2(i)*Lmd(i)^3 - Lmd(i)^3*Lssd(i) - 2*Lfd(i)*Lmd(i)^3 + Lfd(i)*Lkd1(i)*Lmd(i)^2 + Lfd(i)*Lkd2(i)*Lmd(i)^2 + Lkd1(i)*Lkd2(i)*Lmd(i)^2 + Lfd(i)*Lmd(i)^2*Lssd(i) + Lkd2(i)*Lmd(i)^2*Lssd(i) - Lfd(i)*Lkd1(i)*Lkd2(i)*Lssd(i))),  + 0,  + (0 + (Lkd1(i)*Lmd(i)^2 + Lkd2(i)*Lmd(i)^2 - Lmd(i)^3 - Lkd1(i)*Lkd2(i)*Lmd(i))/(2*Lmd(i)^4 - Lkd1(i)*Lmd(i)^3 - 2*Lkd2(i)*Lmd(i)^3 - Lmd(i)^3*Lssd(i) - 2*Lfd(i)*Lmd(i)^3 + Lfd(i)*Lkd1(i)*Lmd(i)^2 + Lfd(i)*Lkd2(i)*Lmd(i)^2 + Lkd1(i)*Lkd2(i)*Lmd(i)^2 + Lfd(i)*Lmd(i)^2*Lssd(i) + Lkd2(i)*Lmd(i)^2*Lssd(i) - Lfd(i)*Lkd1(i)*Lkd2(i)*Lssd(i))),  + (0 + (Lfd(i)*Lmd(i)^2 + Lkd2(i)*Lmd(i)^2 - Lmd(i)^3 - Lfd(i)*Lkd2(i)*Lmd(i))/(2*Lmd(i)^4 - Lkd1(i)*Lmd(i)^3 - 2*Lkd2(i)*Lmd(i)^3 - Lmd(i)^3*Lssd(i) - 2*Lfd(i)*Lmd(i)^3 + Lfd(i)*Lkd1(i)*Lmd(i)^2 + Lfd(i)*Lkd2(i)*Lmd(i)^2 + Lkd1(i)*Lkd2(i)*Lmd(i)^2 + Lfd(i)*Lmd(i)^2*Lssd(i) + Lkd2(i)*Lmd(i)^2*Lssd(i) - Lfd(i)*Lkd1(i)*Lkd2(i)*Lssd(i))),  + (0 + (Lfd(i)*Lmd(i)^2 - Lfd(i)*Lkd1(i)*Lmd(i))/(2*Lmd(i)^4 - Lkd1(i)*Lmd(i)^3 - 2*Lkd2(i)*Lmd(i)^3 - Lmd(i)^3*Lssd(i) - 2*Lfd(i)*Lmd(i)^3 + Lfd(i)*Lkd1(i)*Lmd(i)^2 + Lfd(i)*Lkd2(i)*Lmd(i)^2 + Lkd1(i)*Lkd2(i)*Lmd(i)^2 + Lfd(i)*Lmd(i)^2*Lssd(i) + Lkd2(i)*Lmd(i)^2*Lssd(i) - Lfd(i)*Lkd1(i)*Lkd2(i)*Lssd(i))),  + 0,  + 0,  + 0, ; 0,  + (0 - (Lkq1(i)*Lmq(i)^2 + Lkq2(i)*Lmq(i)^2 + Lkq3(i)*Lmq(i)^2 - 2*Lmq(i)^3 - Lkq1(i)*Lkq2(i)*Lkq3(i))/(3*Lmq(i)^4 - 2*Lkq2(i)*Lmq(i)^3 - 2*Lkq3(i)*Lmq(i)^3 - 2*Lmq(i)^3*Lssq(i) - 2*Lkq1(i)*Lmq(i)^3 + Lkq1(i)*Lkq2(i)*Lmq(i)^2 + Lkq1(i)*Lkq3(i)*Lmq(i)^2 + Lkq2(i)*Lkq3(i)*Lmq(i)^2 + Lkq1(i)*Lmq(i)^2*Lssq(i) + Lkq2(i)*Lmq(i)^2*Lssq(i) + Lkq3(i)*Lmq(i)^2*Lssq(i) - Lkq1(i)*Lkq2(i)*Lkq3(i)*Lssq(i))),  + 0,  + 0,  + 0,  + (0 - (3*Lmq(i)^3 - 2*Lkq2(i)*Lmq(i)^2 - 2*Lkq3(i)*Lmq(i)^2 - 2*Lkq1(i)*Lmq(i)^2 + Lkq1(i)*Lkq2(i)*Lmq(i) + Lkq1(i)*Lkq3(i)*Lmq(i) + Lkq2(i)*Lkq3(i)*Lmq(i))/(3*Lmq(i)^4 - 2*Lkq2(i)*Lmq(i)^3 - 2*Lkq3(i)*Lmq(i)^3 - 2*Lmq(i)^3*Lssq(i) - 2*Lkq1(i)*Lmq(i)^3 + Lkq1(i)*Lkq2(i)*Lmq(i)^2 + Lkq1(i)*Lkq3(i)*Lmq(i)^2 + Lkq2(i)*Lkq3(i)*Lmq(i)^2 + Lkq1(i)*Lmq(i)^2*Lssq(i) + Lkq2(i)*Lmq(i)^2*Lssq(i) + Lkq3(i)*Lmq(i)^2*Lssq(i) - Lkq1(i)*Lkq2(i)*Lkq3(i)*Lssq(i))),  + 0,  + 0, ; (0 - (Lkd2(i)*Lmd(i)^2 - Lkd1(i)*Lkd2(i)*Lmd(i))/(2*Lmd(i)^4 - Lkd1(i)*Lmd(i)^3 - 2*Lkd2(i)*Lmd(i)^3 - Lmd(i)^3*Lssd(i) - 2*Lfd(i)*Lmd(i)^3 + Lfd(i)*Lkd1(i)*Lmd(i)^2 + Lfd(i)*Lkd2(i)*Lmd(i)^2 + Lkd1(i)*Lkd2(i)*Lmd(i)^2 + Lfd(i)*Lmd(i)^2*Lssd(i) + Lkd2(i)*Lmd(i)^2*Lssd(i) - Lfd(i)*Lkd1(i)*Lkd2(i)*Lssd(i))),  + 0,  + (0 + (Lkd1(i)*Lmd(i)^2 + Lkd2(i)*Lmd(i)^2 + Lmd(i)^2*Lssd(i) - 2*Lmd(i)^3 - Lkd1(i)*Lkd2(i)*Lssd(i))/(2*Lmd(i)^4 - Lkd1(i)*Lmd(i)^3 - 2*Lkd2(i)*Lmd(i)^3 - Lmd(i)^3*Lssd(i) - 2*Lfd(i)*Lmd(i)^3 + Lfd(i)*Lkd1(i)*Lmd(i)^2 + Lfd(i)*Lkd2(i)*Lmd(i)^2 + Lkd1(i)*Lkd2(i)*Lmd(i)^2 + Lfd(i)*Lmd(i)^2*Lssd(i) + Lkd2(i)*Lmd(i)^2*Lssd(i) - Lfd(i)*Lkd1(i)*Lkd2(i)*Lssd(i))),  + (0 - (Lkd2(i)*Lmd(i)^2 - Lkd2(i)*Lssd(i)*Lmd(i))/(2*Lmd(i)^4 - Lkd1(i)*Lmd(i)^3 - 2*Lkd2(i)*Lmd(i)^3 - Lmd(i)^3*Lssd(i) - 2*Lfd(i)*Lmd(i)^3 + Lfd(i)*Lkd1(i)*Lmd(i)^2 + Lfd(i)*Lkd2(i)*Lmd(i)^2 + Lkd1(i)*Lkd2(i)*Lmd(i)^2 + Lfd(i)*Lmd(i)^2*Lssd(i) + Lkd2(i)*Lmd(i)^2*Lssd(i) - Lfd(i)*Lkd1(i)*Lkd2(i)*Lssd(i))),  + (0 - (Lkd1(i)*Lmd(i)^2 + Lmd(i)^2*Lssd(i) - 2*Lmd(i)^3)/(2*Lmd(i)^4 - Lkd1(i)*Lmd(i)^3 - 2*Lkd2(i)*Lmd(i)^3 - Lmd(i)^3*Lssd(i) - 2*Lfd(i)*Lmd(i)^3 + Lfd(i)*Lkd1(i)*Lmd(i)^2 + Lfd(i)*Lkd2(i)*Lmd(i)^2 + Lkd1(i)*Lkd2(i)*Lmd(i)^2 + Lfd(i)*Lmd(i)^2*Lssd(i) + Lkd2(i)*Lmd(i)^2*Lssd(i) - Lfd(i)*Lkd1(i)*Lkd2(i)*Lssd(i))),  + 0,  + 0,  + 0, ; (0 - (Lfd(i)*Lmd(i)^2 + Lkd2(i)*Lmd(i)^2 - Lmd(i)^3 - Lfd(i)*Lkd2(i)*Lmd(i))/(2*Lmd(i)^4 - Lkd1(i)*Lmd(i)^3 - 2*Lkd2(i)*Lmd(i)^3 - Lmd(i)^3*Lssd(i) - 2*Lfd(i)*Lmd(i)^3 + Lfd(i)*Lkd1(i)*Lmd(i)^2 + Lfd(i)*Lkd2(i)*Lmd(i)^2 + Lkd1(i)*Lkd2(i)*Lmd(i)^2 + Lfd(i)*Lmd(i)^2*Lssd(i) + Lkd2(i)*Lmd(i)^2*Lssd(i) - Lfd(i)*Lkd1(i)*Lkd2(i)*Lssd(i))),  + 0,  + (0 - (Lkd2(i)*Lmd(i)^2 + Lmd(i)^2*Lssd(i) - Lmd(i)^3 - Lkd2(i)*Lmd(i)*Lssd(i))/(2*Lmd(i)^4 - Lkd1(i)*Lmd(i)^3 - 2*Lkd2(i)*Lmd(i)^3 - Lmd(i)^3*Lssd(i) - 2*Lfd(i)*Lmd(i)^3 + Lfd(i)*Lkd1(i)*Lmd(i)^2 + Lfd(i)*Lkd2(i)*Lmd(i)^2 + Lkd1(i)*Lkd2(i)*Lmd(i)^2 + Lfd(i)*Lmd(i)^2*Lssd(i) + Lkd2(i)*Lmd(i)^2*Lssd(i) - Lfd(i)*Lkd1(i)*Lkd2(i)*Lssd(i))),  + (0 + (Lfd(i)*Lmd(i)^2 + Lkd2(i)*Lmd(i)^2 - Lmd(i)^3 - Lfd(i)*Lkd2(i)*Lssd(i))/(2*Lmd(i)^4 - Lkd1(i)*Lmd(i)^3 - 2*Lkd2(i)*Lmd(i)^3 - Lmd(i)^3*Lssd(i) - 2*Lfd(i)*Lmd(i)^3 + Lfd(i)*Lkd1(i)*Lmd(i)^2 + Lfd(i)*Lkd2(i)*Lmd(i)^2 + Lkd1(i)*Lkd2(i)*Lmd(i)^2 + Lfd(i)*Lmd(i)^2*Lssd(i) + Lkd2(i)*Lmd(i)^2*Lssd(i) - Lfd(i)*Lkd1(i)*Lkd2(i)*Lssd(i))),  + (0 - (Lfd(i)*Lmd(i)^2 - Lfd(i)*Lssd(i)*Lmd(i))/(2*Lmd(i)^4 - Lkd1(i)*Lmd(i)^3 - 2*Lkd2(i)*Lmd(i)^3 - Lmd(i)^3*Lssd(i) - 2*Lfd(i)*Lmd(i)^3 + Lfd(i)*Lkd1(i)*Lmd(i)^2 + Lfd(i)*Lkd2(i)*Lmd(i)^2 + Lkd1(i)*Lkd2(i)*Lmd(i)^2 + Lfd(i)*Lmd(i)^2*Lssd(i) + Lkd2(i)*Lmd(i)^2*Lssd(i) - Lfd(i)*Lkd1(i)*Lkd2(i)*Lssd(i))),  + 0,  + 0,  + 0, ; (0 - (Lfd(i)*Lmd(i)^2 + Lkd1(i)*Lmd(i)^2 - Lmd(i)^3 - Lfd(i)*Lkd1(i)*Lmd(i))/(2*Lmd(i)^4 - Lkd1(i)*Lmd(i)^3 - 2*Lkd2(i)*Lmd(i)^3 - Lmd(i)^3*Lssd(i) - 2*Lfd(i)*Lmd(i)^3 + Lfd(i)*Lkd1(i)*Lmd(i)^2 + Lfd(i)*Lkd2(i)*Lmd(i)^2 + Lkd1(i)*Lkd2(i)*Lmd(i)^2 + Lfd(i)*Lmd(i)^2*Lssd(i) + Lkd2(i)*Lmd(i)^2*Lssd(i) - Lfd(i)*Lkd1(i)*Lkd2(i)*Lssd(i))),  + 0,  + (0 - (Lkd1(i)*Lmd(i)^2 + Lmd(i)^2*Lssd(i) - Lmd(i)^3 - Lkd1(i)*Lmd(i)*Lssd(i))/(2*Lmd(i)^4 - Lkd1(i)*Lmd(i)^3 - 2*Lkd2(i)*Lmd(i)^3 - Lmd(i)^3*Lssd(i) - 2*Lfd(i)*Lmd(i)^3 + Lfd(i)*Lkd1(i)*Lmd(i)^2 + Lfd(i)*Lkd2(i)*Lmd(i)^2 + Lkd1(i)*Lkd2(i)*Lmd(i)^2 + Lfd(i)*Lmd(i)^2*Lssd(i) + Lkd2(i)*Lmd(i)^2*Lssd(i) - Lfd(i)*Lkd1(i)*Lkd2(i)*Lssd(i))),  + (0 - (Lfd(i)*Lmd(i)^2 + Lmd(i)^2*Lssd(i) - Lmd(i)^3 - Lfd(i)*Lmd(i)*Lssd(i))/(2*Lmd(i)^4 - Lkd1(i)*Lmd(i)^3 - 2*Lkd2(i)*Lmd(i)^3 - Lmd(i)^3*Lssd(i) - 2*Lfd(i)*Lmd(i)^3 + Lfd(i)*Lkd1(i)*Lmd(i)^2 + Lfd(i)*Lkd2(i)*Lmd(i)^2 + Lkd1(i)*Lkd2(i)*Lmd(i)^2 + Lfd(i)*Lmd(i)^2*Lssd(i) + Lkd2(i)*Lmd(i)^2*Lssd(i) - Lfd(i)*Lkd1(i)*Lkd2(i)*Lssd(i))),  + (0 + (Lfd(i)*Lmd(i)^2 + Lkd1(i)*Lmd(i)^2 + Lmd(i)^2*Lssd(i) - 2*Lmd(i)^3 - Lfd(i)*Lkd1(i)*Lssd(i))/(2*Lmd(i)^4 - Lkd1(i)*Lmd(i)^3 - 2*Lkd2(i)*Lmd(i)^3 - Lmd(i)^3*Lssd(i) - 2*Lfd(i)*Lmd(i)^3 + Lfd(i)*Lkd1(i)*Lmd(i)^2 + Lfd(i)*Lkd2(i)*Lmd(i)^2 + Lkd1(i)*Lkd2(i)*Lmd(i)^2 + Lfd(i)*Lmd(i)^2*Lssd(i) + Lkd2(i)*Lmd(i)^2*Lssd(i) - Lfd(i)*Lkd1(i)*Lkd2(i)*Lssd(i))),  + 0,  + 0,  + 0, ; 0,  + (0 - (Lkq2(i)*Lmq(i)^2 + Lkq3(i)*Lmq(i)^2 - Lmq(i)^3 - Lkq2(i)*Lkq3(i)*Lmq(i))/(3*Lmq(i)^4 - 2*Lkq2(i)*Lmq(i)^3 - 2*Lkq3(i)*Lmq(i)^3 - 2*Lmq(i)^3*Lssq(i) - 2*Lkq1(i)*Lmq(i)^3 + Lkq1(i)*Lkq2(i)*Lmq(i)^2 + Lkq1(i)*Lkq3(i)*Lmq(i)^2 + Lkq2(i)*Lkq3(i)*Lmq(i)^2 + Lkq1(i)*Lmq(i)^2*Lssq(i) + Lkq2(i)*Lmq(i)^2*Lssq(i) + Lkq3(i)*Lmq(i)^2*Lssq(i) - Lkq1(i)*Lkq2(i)*Lkq3(i)*Lssq(i))),  + 0,  + 0,  + 0,  + (0 - (Lmq(i)^2*Lssq(i) + Lkq2(i)*Lkq3(i)*Lssq(i) - Lkq2(i)*Lmq(i)*Lssq(i) - Lkq3(i)*Lmq(i)*Lssq(i))/(3*Lmq(i)^4 - 2*Lkq2(i)*Lmq(i)^3 - 2*Lkq3(i)*Lmq(i)^3 - 2*Lmq(i)^3*Lssq(i) - 2*Lkq1(i)*Lmq(i)^3 + Lkq1(i)*Lkq2(i)*Lmq(i)^2 + Lkq1(i)*Lkq3(i)*Lmq(i)^2 + Lkq2(i)*Lkq3(i)*Lmq(i)^2 + Lkq1(i)*Lmq(i)^2*Lssq(i) + Lkq2(i)*Lmq(i)^2*Lssq(i) + Lkq3(i)*Lmq(i)^2*Lssq(i) - Lkq1(i)*Lkq2(i)*Lkq3(i)*Lssq(i))),  + 0,  + 0, ; 0,  + (0 + (Lmq(i)*(Lkq1(i) - Lmq(i))*(Lkq3(i) - Lmq(i)))/(3*Lmq(i)^4 - 2*Lkq2(i)*Lmq(i)^3 - 2*Lkq3(i)*Lmq(i)^3 - 2*Lmq(i)^3*Lssq(i) - 2*Lkq1(i)*Lmq(i)^3 + Lkq1(i)*Lkq2(i)*Lmq(i)^2 + Lkq1(i)*Lkq3(i)*Lmq(i)^2 + Lkq2(i)*Lkq3(i)*Lmq(i)^2 + Lkq1(i)*Lmq(i)^2*Lssq(i) + Lkq2(i)*Lmq(i)^2*Lssq(i) + Lkq3(i)*Lmq(i)^2*Lssq(i) - Lkq1(i)*Lkq2(i)*Lkq3(i)*Lssq(i))),  + 0,  + 0,  + 0,  + (0 - (Lssq(i)*(Lkq1(i) - Lmq(i))*(Lkq3(i) - Lmq(i)))/(3*Lmq(i)^4 - 2*Lkq2(i)*Lmq(i)^3 - 2*Lkq3(i)*Lmq(i)^3 - 2*Lmq(i)^3*Lssq(i) - 2*Lkq1(i)*Lmq(i)^3 + Lkq1(i)*Lkq2(i)*Lmq(i)^2 + Lkq1(i)*Lkq3(i)*Lmq(i)^2 + Lkq2(i)*Lkq3(i)*Lmq(i)^2 + Lkq1(i)*Lmq(i)^2*Lssq(i) + Lkq2(i)*Lmq(i)^2*Lssq(i) + Lkq3(i)*Lmq(i)^2*Lssq(i) - Lkq1(i)*Lkq2(i)*Lkq3(i)*Lssq(i))),  + 0,  + 0, ; 0,  + (0 + (Lmq(i)*(Lkq1(i) - Lmq(i))*(Lkq2(i) - Lmq(i)))/(3*Lmq(i)^4 - 2*Lkq2(i)*Lmq(i)^3 - 2*Lkq3(i)*Lmq(i)^3 - 2*Lmq(i)^3*Lssq(i) - 2*Lkq1(i)*Lmq(i)^3 + Lkq1(i)*Lkq2(i)*Lmq(i)^2 + Lkq1(i)*Lkq3(i)*Lmq(i)^2 + Lkq2(i)*Lkq3(i)*Lmq(i)^2 + Lkq1(i)*Lmq(i)^2*Lssq(i) + Lkq2(i)*Lmq(i)^2*Lssq(i) + Lkq3(i)*Lmq(i)^2*Lssq(i) - Lkq1(i)*Lkq2(i)*Lkq3(i)*Lssq(i))),  + 0,  + 0,  + 0,  + (0 - (Lssq(i)*(Lkq1(i) - Lmq(i))*(Lkq2(i) - Lmq(i)))/(3*Lmq(i)^4 - 2*Lkq2(i)*Lmq(i)^3 - 2*Lkq3(i)*Lmq(i)^3 - 2*Lmq(i)^3*Lssq(i) - 2*Lkq1(i)*Lmq(i)^3 + Lkq1(i)*Lkq2(i)*Lmq(i)^2 + Lkq1(i)*Lkq3(i)*Lmq(i)^2 + Lkq2(i)*Lkq3(i)*Lmq(i)^2 + Lkq1(i)*Lmq(i)^2*Lssq(i) + Lkq2(i)*Lmq(i)^2*Lssq(i) + Lkq3(i)*Lmq(i)^2*Lssq(i) - Lkq1(i)*Lkq2(i)*Lkq3(i)*Lssq(i))),  + 0,  + 0, ];
      |     end
  isd : Outport
  isq : Outport  Port=2
  psi : Outport  Port=3

== system VFlexP/Grid/Generators/SG/For Each Subsystem ==
  In1 : Inport  Partition=on  PartitionDimension=1  PartitionWidth=1  PartitionOffset=0
  For Each : ForEach  DisableCoverage=on
  State-Space : StateSpace  A=[]  B=[]  C=[]  D=block_toM  InitialCondition=0  ParameterTunability=Optimized
  Transpose : Math  Operator=transpose
  Transpose1 : Math  Operator=transpose
  Out1 : Outport  ConcatenationDimension=1
  wires:
  Transpose1/1 -> Out1/1
  In1/1 -> Transpose/1
  Transpose/1 -> State-Space/1
  State-Space/1 -> Transpose1/1

== system VFlexP/Grid/Generators/SG/LPF2 ==
  in : Inport
  Gain : Gain  Gain=1./T_s
  Sum4 : Sum  Inputs=|+-
  x_a : Integrator  InitialCondition=Grid_op_SG.op.States(4).x'
  out : Outport
  wires:
  Gain/1 -> x_a/1
  Sum4/1 -> Gain/1
  in/1 -> Sum4/1
  x_a/1 -> out/1, Sum4/2

== system VFlexP/Grid/Generators/SG/LPF4 ==
  in : Inport
  Gain : Gain  Gain=1./T_s
  Sum4 : Sum  Inputs=|+-
  x_a : Integrator  InitialCondition=Grid_op_SG.op.States(10).x'
  out : Outport
  wires:
  x_a/1 -> Sum4/2, out/1
  in/1 -> Sum4/1
  Sum4/1 -> Gain/1
  Gain/1 -> x_a/1

== system VFlexP/Grid/Generators/SG/LPF5 ==
  in : Inport
  Gain : Gain  Gain=1./T_s
  Sum4 : Sum  Inputs=|+-
  x_a : Integrator  InitialCondition=Grid_op_SG.op.States(11).x'
  out : Outport
  wires:
  Gain/1 -> x_a/1
  Sum4/1 -> Gain/1
  in/1 -> Sum4/1
  x_a/1 -> out/1, Sum4/2

== system VFlexP/Grid/Generators/SG/PIv_d1 ==
  In1 : Inport
  Gain : Gain  Gain=10
  Gain1 : Gain  Gain=200
  I : Integrator  InitialCondition=Grid_op_SG.op.States(7).x'
  Sum10 : Sum  Inputs=|++
  vfd : Outport
  wires:
  In1/1 -> Gain1/1, Gain/1
  Sum10/1 -> vfd/1
  Gain/1 -> Sum10/1
  I/1 -> Sum10/2
  Gain1/1 -> I/1

== system VFlexP/Grid/Generators/SG/Reference frame transform1 ==
  in_d : Inport
  theta : Inport  Port=2
  in_q : Inport  Port=3
  Complex to Real-Imag : ComplexToRealImag
  Cos : Trigonometry  SCDEnableBlockLinearizationSpecification=on  Operator=cos
  Product : Product
  Real-Imag to Complex : RealImagToComplex
  Real-Imag to Complex1 : RealImagToComplex
  Sin : Trigonometry  SCDEnableBlockLinearizationSpecification=on
  out_d : Outport
  out_q : Outport  Port=2
  wires:
  in_d/1 -> Real-Imag to Complex/1
  in_q/1 -> Real-Imag to Complex/2
  Complex to Real-Imag/1 -> out_d/1
  Sin/1 -> Real-Imag to Complex1/2
  Cos/1 -> Real-Imag to Complex1/1
  theta/1 -> Cos/1, Sin/1
  Product/1 -> Complex to Real-Imag/1
  Real-Imag to Complex/1 -> Product/2
  Real-Imag to Complex1/1 -> Product/1
  Complex to Real-Imag/2 -> out_q/1

== system VFlexP/Grid/Generators/SG/Reference frame transform3 ==
  in_d : Inport
  theta : Inport  Port=2
  in_q : Inport  Port=3
  Complex to Real-Imag : ComplexToRealImag
  Cos : Trigonometry  SCDEnableBlockLinearizationSpecification=on  Operator=cos
  Product : Product
  Real-Imag to Complex : RealImagToComplex
  Real-Imag to Complex1 : RealImagToComplex
  Sin : Trigonometry  SCDEnableBlockLinearizationSpecification=on
  out_d : Outport
  out_q : Outport  Port=2
  wires:
  Complex to Real-Imag/2 -> out_q/1
  Real-Imag to Complex1/1 -> Product/1
  Real-Imag to Complex/1 -> Product/2
  Product/1 -> Complex to Real-Imag/1
  theta/1 -> Sin/1, Cos/1
  Cos/1 -> Real-Imag to Complex1/1
  Sin/1 -> Real-Imag to Complex1/2
  Complex to Real-Imag/1 -> out_d/1
  in_q/1 -> Real-Imag to Complex/2
  in_d/1 -> Real-Imag to Complex/1

== system VFlexP/Grid/Generators/SG/Rotor axis ==
  te : Inport
  tm : Inport  Port=2
  Gain : Gain  Gain=1/2./H
  Gain1 : Gain  Gain=D
  Sum1 : Sum  Inputs=+|-|-  InputSameDT=on  SaturateOnIntegerOverflow=on  OutDataTypeStr=Inherit: Same as first input
  \omega_r : Integrator  InitialCondition=Grid_op_SG.op.States(7).x'  UpperSaturationLimit=2*pi  LowerSaturationLimit=0
  wr : Outport  VectorParamsAs1DForOutWhenUnconnected=off
  wires:
  tm/1 -> Sum1/1
  \omega_r/1 -> wr/1, Gain1/1
  te/1 -> Sum1/2
  Sum1/1 -> Gain/1
  Gain/1 -> \omega_r/1
  Gain1/1 -> Sum1/3

== system VFlexP/Grid/Generators/SG/Subsystem2 ==
  In1 : Inport
  Gain : Gain  Gain=1./T_1
  Gain2 : Gain  Gain=T_2./T_1
  Sum : Sum  Inputs=|+-
  Sum1 : Sum  Inputs=++|
  x_f : Integrator  InitialCondition=Grid_op_SG.op.States(17).x'
  Out1 : Outport
  wires:
  x_f/1 -> Sum1/2, Sum/2
  Gain/1 -> x_f/1
  Sum/1 -> Gain/1, Gain2/1
  Gain2/1 -> Sum1/1
  Sum1/1 -> Out1/1
  In1/1 -> Sum/1

== system VFlexP/Grid/Generators/SG/Subsystem4 ==
  In1 : Inport
  Gain : Gain  Gain=1./T_1
  Gain2 : Gain  Gain=T_2./T_1
  Sum : Sum  Inputs=|+-
  Sum1 : Sum  Inputs=++|
  x_f : Integrator  InitialCondition=Grid_op_SG.op.States(18).x'
  Out1 : Outport
  wires:
  x_f/1 -> Sum1/2, Sum/2
  Gain/1 -> x_f/1
  Sum/1 -> Gain/1, Gain2/1
  Gain2/1 -> Sum1/1
  Sum1/1 -> Out1/1
  In1/1 -> Sum/1

== system VFlexP/Grid/Generators/SG/Torque ==
  psi : Inport
  isd : Inport  Port=2
  isq : Inport  Port=3
  Product1 : Product
  Product2 : Product
  Selector : Selector  NumberOfDimensions=2  InputPortWidth=9  IndexOptions=Index vector (dialog),Select all  Indices=[1],1  OutputSizes=1,1
  Selector1 : Selector  NumberOfDimensions=2  InputPortWidth=9  IndexOptions=Index vector (dialog),Select all  Indices=[2],1  OutputSizes=1,1
  Sum : Sum  Inputs=+||-
  te : Outport  VectorParamsAs1DForOutWhenUnconnected=off
  wires:
  Product1/1 -> Sum/1
  Sum/1 -> te/1
  Selector/1 -> Product1/1  "psistatordq"
  psi/1 -> Selector1/1, Selector/1
  Product2/1 -> Sum/2
  isq/1 -> Product1/2
  isd/1 -> Product2/1
  Selector1/1 -> Product2/2  "psistatordq"

== system VFlexP/Grid/Generators/SG/connect ==
  id : Inport
  iq : Inport  Port=2
  connect : Inport  Port=3
  Switch : Switch  Criteria=u2 > Threshold  ZeroCross=off  SaturateOnIntegerOverflow=off  InputSameDT=off
  Switch1 : Switch  Criteria=u2 > Threshold  ZeroCross=off  SaturateOnIntegerOverflow=off  InputSameDT=off
  Zero1 : Constant  Value=0  VectorParams1D=off  OutDataTypeStr=Inherit: Inherit via back propagation
  Zero2 : Constant  Value=0  VectorParams1D=off  OutDataTypeStr=Inherit: Inherit via back propagation
  id_real : Outport
  iq_real : Outport  Port=2
  connected : Outport  Port=3  OutDataTypeStr=boolean
  wires:
  Switch/1 -> id_real/1
  Zero1/1 -> Switch/3
  id/1 -> Switch/1
  connect/1 -> connected/1, Switch1/2, Switch/2
  Switch1/1 -> iq_real/1
  iq/1 -> Switch1/1
  Zero2/1 -> Switch1/3

== system VFlexP/Grid/Generators/SG/trim_output ==
  id : Inport
  iq : Inport  Port=2
  vd : Inport  Port=3
  vq : Inport  Port=4
  Out1 : Outport
  Out2 : Outport  Port=2
  Out3 : Outport  Port=3
  Out4 : Outport  Port=4
  wires:
  id/1 -> Out1/1
  vq/1 -> Out4/1
  vd/1 -> Out3/1
  iq/1 -> Out2/1

== system VFlexP/Grid/Generators/VSM/For Each Subsystem ==
  In1 : Inport  Partition=on  PartitionDimension=1  PartitionWidth=1  PartitionOffset=0
  For Each : ForEach  DisableCoverage=on
  State-Space : StateSpace  A=[]  B=[]  C=[]  D=block_toM  InitialCondition=0  ParameterTunability=Optimized
  Transpose : Math  Operator=transpose
  Transpose1 : Math  Operator=transpose
  Out1 : Outport  ConcatenationDimension=1
  wires:
  In1/1 -> Transpose/1
  Transpose1/1 -> Out1/1
  Transpose/1 -> State-Space/1
  State-Space/1 -> Transpose1/1

== system VFlexP/Grid/Generators/VSM/LPF1 ==
  In1 : Inport
  Gain : Gain  Gain=1e2
  I : Integrator  InitialCondition=Grid_op_VSM.op.States(2).x'
  Sum4 : Sum  Inputs=|+-
  Out1 : Outport
  wires:
  I/1 -> Sum4/2, Out1/1
  In1/1 -> Sum4/1
  Sum4/1 -> Gain/1
  Gain/1 -> I/1

== system VFlexP/Grid/Generators/VSM/LPF4 ==
  In1 : Inport
  Gain : Gain  Gain=1e2
  I : Integrator  InitialCondition=Grid_op_VSM.op.States(3).x'
  Sum4 : Sum  Inputs=|+-
  Out1 : Outport
  wires:
  Gain/1 -> I/1
  Sum4/1 -> Gain/1
  In1/1 -> Sum4/1
  I/1 -> Out1/1, Sum4/2

== system VFlexP/Grid/Generators/VSM/LPF5 ==
  In1 : Inport
  Gain : Gain  Gain=1e2
  I : Integrator  InitialCondition=Grid_op_VSM.op.States(4).x'
  Sum4 : Sum  Inputs=|+-
  Out1 : Outport
  wires:
  I/1 -> Sum4/2, Out1/1
  In1/1 -> Sum4/1
  Sum4/1 -> Gain/1
  Gain/1 -> I/1
